simulink model "full_sim123deleteme"  (R2020b)
settings: Solver=ode1be  StartTime=0.0  StopTime=inf  RelTol=1e-3
InitFcn:
  | % Clear persistent variables in callback
  | clear all;
  | 
  | track = gen_track;
  | map = double(rgb2gray(imread('map.png')));%'iSpaceMapV2.0_50dpi.png')))*100/255;
  | 
  | % Load config data automatically
  | load("config.mat");
StartFcn:
  | % The event listener triggers when the signal updates, so we can just monitor one of the signals.
  | blk1 = 'full_sim/GUI_update';
  | 
  | event = 'PostOutputs';
  | listener = @updateApp;
  | 
  | % Create the listener
  | h1 = add_exec_event_listener(blk1, event, listener);
model workspace (MAT data in the model file):
  ResetMode = "Reset at each sample time"
  initX = -0.39
  initY = 0.33
  initYaw = 3.14159265359
libraries: simulink_extras x10, simulink x8, dspnetwork x6, pid_lib x2, sldrtlib x1
(part 1 of 2)
settings Model: Creator=Duncan  LastModifiedBy=dffleiss

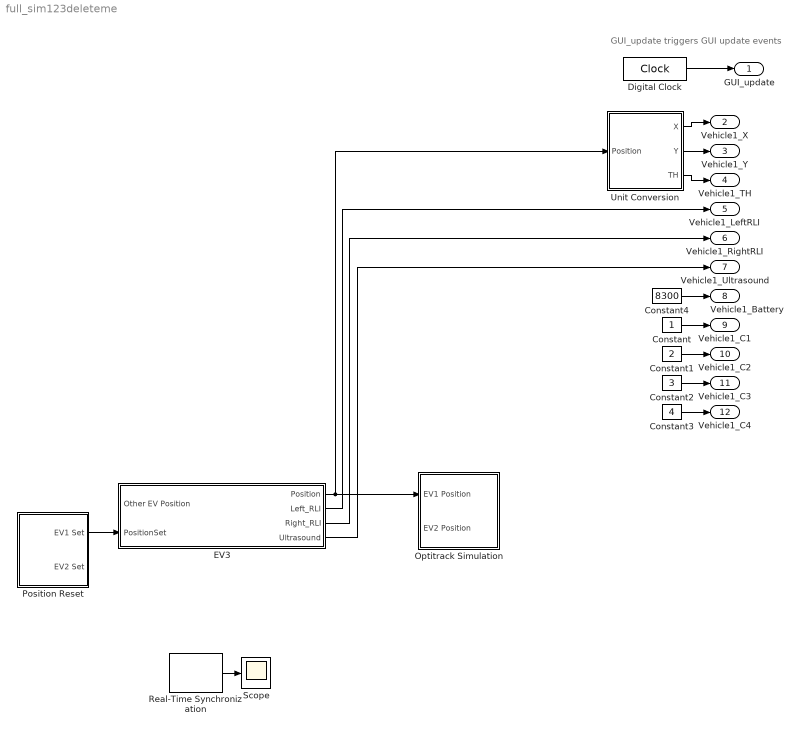
== system full_sim123deleteme ==
  note: GUI_update triggers GUI update events
  Constant : Constant
  Constant1 : Constant  Value=2
  Constant2 : Constant  Value=3
  Constant3 : Constant  Value=4
  Constant4 : Constant  Value=8300
  Digital Clock : DigitalClock  SampleTime=0.1
  EV3 : Subsystem
  Optitrack Simulation : Subsystem
  Position Reset : Subsystem
  Real-Time Synchronization : sldrtlib/Real-Time Synchronization  SampleTime=.01  MaxMissedTicks=inf  ShowMissedTicks=on  YieldWhenWaiting=off
  Scope : Scope
  Unit Conversion : Subsystem
  GUI_update : Outport
  Vehicle1_X : Outport  Port=2
  Vehicle1_Y : Outport  Port=3
  Vehicle1_TH : Outport  Port=4
  Vehicle1_LeftRLI : Outport  Port=5
  Vehicle1_RightRLI : Outport  Port=6
  Vehicle1_Ultrasound : Outport  Port=7
  Vehicle1_Battery : Outport  Port=8
  Vehicle1_C1 : Outport  Port=9
  Vehicle1_C2 : Outport  Port=10
  Vehicle1_C3 : Outport  Port=11
  Vehicle1_C4 : Outport  Port=12
  wires:
  Real-Time Synchronization/1 -> Scope/1
  Position Reset/1(EV1 Set) -> EV3/2(PositionSet)
  Constant2/1 -> Vehicle1_C3/1
  Constant4/1 -> Vehicle1_Battery/1
  Constant1/1 -> Vehicle1_C2/1
  EV3/2(Left_RLI) -> Vehicle1_LeftRLI/1
  Constant/1 -> Vehicle1_C1/1
  Constant3/1 -> Vehicle1_C4/1
  EV3/1(Position) -> Unit Conversion/1(Position), Optitrack Simulation/1(EV1 Position)
  Unit Conversion/2(Y) -> Vehicle1_Y/1
  Unit Conversion/3(TH) -> Vehicle1_TH/1
  Unit Conversion/1(X) -> Vehicle1_X/1
  Digital Clock/1 -> GUI_update/1
  EV3/3(Right_RLI) -> Vehicle1_RightRLI/1
  EV3/4(Ultrasound) -> Vehicle1_Ultrasound/1

== system full_sim123deleteme/EV3 ==
  Other EV Position : Inport
  PositionSet : Inport  Port=2
  Additive Noise : Subsystem
  Localization and UI Control : Subsystem
      settings: PortSchema="{\"entries\":[{\"content\":{\"sides\":[{\"content\":{\"connectorIds\":[\"Out1\",\"Out2\"]},\"type\":\"ConnectorPlacement.EquallySpacedRectSide\",\"uuid\":\"c41f9887-e70f-42cb-a70d-ce479c94e8e6\"},{\"content\":{\"connectorIds\":[\"In7\",\"In8\",\"In9\"],\"side\":\"RIGHT\"},\"type\":\"ConnectorPlacement.EquallySpacedRectSide\",\"uuid\":\"01fea69d-4e07-40c9-8b78-412f64609b36\"},{\"content\":{\"connectorIds\":[\"In1\",\"In2\",\"In3\",\"In4\",\"In5\",\"In6\"],\"side\":\"TOP\"},\"type\":\"ConnectorPlacement.EquallySpacedRectSide\",\"uuid\":\"d2fc7682-afac-46c9-9372-ea085883672c\"}]},\"type\":\"ConnectorPlacement.EquallySpacedConnector\",\"uuid\":\"f49fd9b7-3a1c-45a5-ac31-ef3904fd2313\"}],\"packageUris\":[\"http://schema.mathworks.com/mf0/Connector/19700101\"],\"version\":\"1.0\"}"
  Position Control : Subsystem
  Sensor Input Block : Subsystem
  Task Controls : Subsystem
      settings: PortSchema="{\"entries\":[{\"content\":{\"sides\":[{\"content\":{\"connectorIds\":[\"In1\",\"In2\",\"In3\",\"In4\",\"In5\"]},\"type\":\"ConnectorPlacement.EquallySpacedRectSide\",\"uuid\":\"3c64813c-625d-49d1-ae67-306451c3c1fa\"},{\"content\":{\"connectorIds\":[\"Out1\",\"Out2\",\"Out3\",\"Out4\"],\"side\":\"RIGHT\"},\"type\":\"ConnectorPlacement.EquallySpacedRectSide\",\"uuid\":\"91793cf5-b7a0-4d71-a2c0-83cdd43afca2\"},{\"content\":{\"connectorIds\":[],\"side\":\"TOP\"},\"type\":\"ConnectorPlacement.EquallySpacedRectSide\",\"uuid\":\"5300aefe-28d7-4142-9759-b53f625cf082\"},{\"content\":{\"connectorIds\":[\"Out5\",\"Out6\",\"Out7\",\"Out8\",\"Out9\",\"Out10\"],\"side\":\"BOTTOM\"},\"type\":\"ConnectorPlacement.EquallySpacedRectSide\",\"uuid\":\"7541b0a2-c079-4b1b-9276-8e4ee5949dfd\"},{\"content\":{\"connectorIds\":[],\"side\":\"HIDDEN\"},\"type\":\"ConnectorPlacement.EquallySpacedRectSide\",\"uuid\":\"d0ef4c96-52b1-4a81-ac1e-c57b650a37a1\"}]},\"type\":\"ConnectorPlacement.EquallySpacedConnector\",\"uuid\":\"d02aae7f-e4d5-4935-81ce-eef5c5855771\"}],\"packageUris\":[\"http://schema.mathworks.com/mf0/Connector/R2020b\"],\"version\":\"1.0\"}"
  Position : Outport
  Left_RLI : Outport  Port=2
  Right_RLI : Outport  Port=3
  Ultrasound : Outport  Port=4
  wires:
  Localization and UI Control/2(Left %) -> Task Controls/4(Left Motor %)
  Position Control/2(Gyro) -> Localization and UI Control/9(Gyro Rate (deg/s))
  Task Controls/2(Right Encoder) -> Localization and UI Control/8(Right Encoder (deg/sample))
  PositionSet/1 -> Position Control/1(Position Set)
  Other EV Position/1 -> Sensor Input Block/2(Other EV Position)
  Position Control/1(Position) -> Position/1, Sensor Input Block/1(Position)
  Localization and UI Control/1(Right %) -> Task Controls/5(Right Motor %)
  Task Controls/1(Left Encoder) -> Localization and UI Control/7(Left Encoder (deg/sample))
  Task Controls/4(Left ω) -> Position Control/3(Input1)
  Task Controls/3(Right ω) -> Position Control/2(Input)
  Task Controls/7(Speed) -> Localization and UI Control/3(LF Speed)
  Task Controls/6(Steering) -> Localization and UI Control/2(LF Steering)
  Task Controls/5(Platoon Speed) -> Localization and UI Control/1(Platoon Speed)
  Task Controls/10(Left RLI) -> Left_RLI/1, Localization and UI Control/6(Left RLI)
  Task Controls/9(Right RLI) -> Right_RLI/1, Localization and UI Control/5(Right RLI)
  Task Controls/8(Ultrasonic) -> Ultrasound/1, Localization and UI Control/4(Ultrasonic (cm))
  Sensor Input Block/1(Left RLI) -> Additive Noise/1(In1)
  Additive Noise/1(Out1) -> Task Controls/1(Left Input)
  Sensor Input Block/2(Right RLI) -> Additive Noise/2(In2)
  Sensor Input Block/3(Ultrasonic) -> Additive Noise/3(In3)
  Additive Noise/2(Out2) -> Task Controls/2(Right Input)
  Additive Noise/3(Out3) -> Task Controls/3(Distance Input)

== system full_sim123deleteme/Optitrack Simulation ==
  EV1 Position : Inport
  EV2 Position : Inport  Port=2
  MATLAB Function : MATLAB Function  TreatAsAtomicUnit=on
  UDP Send : dspnetwork/UDP Send  remoteURL='127.0.0.1'  remotePort=1511  localURL='0.0.0.0'  localPortSource=Automatically determine  localPort=-1  sendBufferSize=8192  sampletime=-1  blockPlatform=[]  separateLengthPort=0
  wires:
  EV1 Position/1 -> MATLAB Function/1(ev1pos)
  EV2 Position/1 -> MATLAB Function/2(ev2pos)
  MATLAB Function/1(packet) -> UDP Send/1

== system full_sim123deleteme/Position Reset ==
  AND : Logic  IconShape=distinctive  AllPortsSameDT=off  OutDataTypeStr=boolean
  AND1 : Logic  IconShape=distinctive  AllPortsSameDT=off  OutDataTypeStr=boolean
  Assignment : Assignment  DiagnosticForDimensions=Warning  IndexOptions=Index vector (dialog)  Indices=1  OutputSizes=1
  Assignment1 : Assignment  DiagnosticForDimensions=Warning  IndexOptions=Index vector (dialog)  Indices=1  OutputSizes=1
  Cast To Single : DataTypeConversion  OutDataTypeStr=single
  Cast To Single1 : DataTypeConversion  OutDataTypeStr=single
  Compare To Constant : simulink/Logic and Bit Operations/Compare To Constant  relop===  const=1  OutDataTypeStr=boolean
  Compare To Constant1 : simulink/Logic and Bit Operations/Compare To Constant  relop===  const=2  OutDataTypeStr=boolean
  Compare To Constant2 : simulink/Logic and Bit Operations/Compare To Constant  relop=>  const=0  OutDataTypeStr=boolean
  UDP Receive : dspnetwork/UDP Receive  localURL='0.0.0.0'  localPort=24999  remoteURL='0.0.0.0'  remotePort=-1  recvBufferSize=512  dims=4  signalDatatype=single  isComplex=off  isVarSize=off  showBlockingTime=off  blockingTime=0  sampletime=0.01  blockPlatform=[]
  ev : Selector  InputPortWidth=4  IndexOptions=Index vector (dialog)  Indices=[1]  OutputSizes=1
  EV1 Set : Outport
  EV2 Set : Outport  Port=2
  wires:
  Compare To Constant2/1 -> AND1/2, AND/2
  UDP Receive/2 -> Compare To Constant2/1
  ev/1 -> Compare To Constant1/1, Compare To Constant/1
  Assignment/1 -> EV1 Set/1
  Compare To Constant/1 -> AND1/1
  Assignment1/1 -> EV2 Set/1
  UDP Receive/1 -> Assignment/1, Assignment1/1, ev/1
  AND/1 -> Cast To Single1/1
  Compare To Constant1/1 -> AND/1
  Cast To Single/1 -> Assignment/2
  AND1/1 -> Cast To Single/1
  Cast To Single1/1 -> Assignment1/2

== system full_sim123deleteme/Unit Conversion ==
  Position : Inport
  Demux1 : Demux  Outputs=3
  Gain2 : Gain  Gain=1000
  Gain3 : Gain  Gain=1000
  MATLAB Function1 : MATLAB Function  TreatAsAtomicUnit=on
  Radians to Degrees1 : simulink_extras/Transformations/Radians to Degrees
  X : Outport
  Y : Outport  Port=2
  TH : Outport  Port=3
  wires:
  Radians to Degrees1/1 -> MATLAB Function1/1(u)
  Gain3/1 -> Y/1
  Demux1/3 -> Radians to Degrees1/1
  Demux1/2 -> Gain3/1
  Gain2/1 -> X/1
  MATLAB Function1/1(y) -> TH/1
  Demux1/1 -> Gain2/1
  Position/1 -> Demux1/1

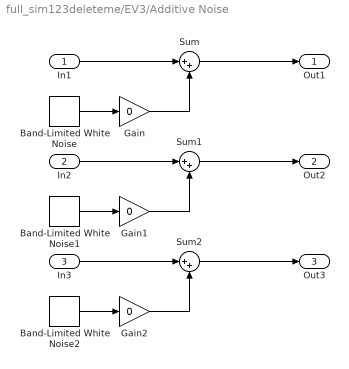
== system full_sim123deleteme/EV3/Additive Noise ==
  In1 : Inport
  In2 : Inport  Port=2
  In3 : Inport  Port=3
  Band-Limited White Noise : simulink/Sources/Band-Limited White Noise  Cov=[0.1]  Ts=0.1  seed=[23341]
  Band-Limited White Noise1 : simulink/Sources/Band-Limited White Noise  Cov=[0.1]  Ts=0.1  seed=[23341]
  Band-Limited White Noise2 : simulink/Sources/Band-Limited White Noise  Cov=[0.1]  Ts=0.1  seed=[23341]
  Gain : Gain  Gain=0
  Gain1 : Gain  Gain=0
  Gain2 : Gain  Gain=0
  Sum : Sum  Inputs=|++
  Sum1 : Sum  Inputs=|++
  Sum2 : Sum  Inputs=|++
  Out1 : Outport
  Out2 : Outport  Port=2
  Out3 : Outport  Port=3
  wires:
  In1/1 -> Sum/1
  Sum/1 -> Out1/1
  Band-Limited White Noise1/1 -> Gain1/1
  Sum1/1 -> Out2/1
  In2/1 -> Sum1/1
  Band-Limited White Noise2/1 -> Gain2/1
  Sum2/1 -> Out3/1
  In3/1 -> Sum2/1
  Band-Limited White Noise/1 -> Gain/1
  Gain/1 -> Sum/2
  Gain1/1 -> Sum1/2
  Gain2/1 -> Sum2/2

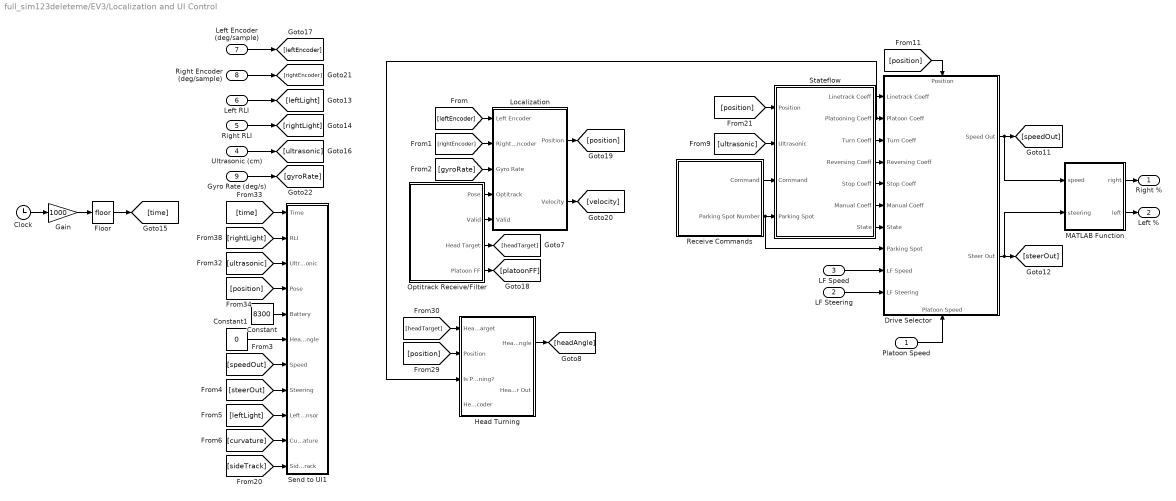
== system full_sim123deleteme/EV3/Localization and UI Control ==
  Platoon Speed : Inport
  LF Steering : Inport  Port=2
  LF Speed : Inport  Port=3
  Ultrasonic (cm) : Inport  Port=4
  Right RLI : Inport  Port=5
  Left RLI : Inport  Port=6
  Left Encoder (deg/sample) : Inport  Port=7
  Right Encoder (deg/sample) : Inport  Port=8
  Gyro Rate (deg/s) : Inport  Port=9
  Clock : Clock
  Constant : Constant  Value=8300
  Constant1 : Constant  Value=0
  Drive Selector : Subsystem
      settings: PortSchema="{\"entries\":[{\"content\":{\"sides\":[{\"content\":{\"connectorIds\":[\"In1\",\"In2\",\"In3\",\"In4\",\"In5\",\"In6\",\"In7\",\"In8\",\"In9\",\"In10\"]},\"type\":\"ConnectorPlacement.EquallySpacedRectSide\",\"uuid\":\"ae307232-287c-4602-bc59-e7aee20cf720\"},{\"content\":{\"connectorIds\":[\"Out1\",\"Out2\"],\"side\":\"RIGHT\"},\"type\":\"ConnectorPlacement.EquallySpacedRectSide\",\"uuid\":\"2cae2544-d808-4029-9530-a1f56251b9cd\"},{\"content\":{\"connectorIds\":[\"In11\"],\"side\":\"TOP\"},\"type\":\"ConnectorPlacement.EquallySpacedRectSide\",\"uuid\":\"bbc0be7b-0147-487e-824e-99eef1e06dcc\"},{\"content\":{\"connectorIds\":[\"In12\"],\"side\":\"BOTTOM\"},\"type\":\"ConnectorPlacement.EquallySpacedRectSide\",\"uuid\":\"b1fbed80-afe2-48db-af11-c85938407aae\"}]},\"type\":\"ConnectorPlacement.EquallySpacedConnector\",\"uuid\":\"38f7d747-6147-4f1b-8575-02c2e0fe0660\"}],\"packageUris\":[\"http://schema.mathworks.com/mf0/Connector/19700101\"],\"version\":\"1.0\"}"
  Floor : Rounding
  Gain : Gain  Gain=1000
  Head Turning : Subsystem
  Localization : Subsystem
  MATLAB Function : MATLAB Function  TreatAsAtomicUnit=on
  Optitrack Receive/Filter : Subsystem
  Receive Commands : Subsystem
  Send to UI1 : Subsystem
  Stateflow : Subsystem
  Right % : Outport
  Left % : Outport  Port=2
  wires:
  Constant/1 -> Send to UI1/5(Battery)
  [position] -> Head Turning/2(Position)
  Left RLI/1 -> [leftLight]
  Localization/2(Velocity) -> [velocity]
  Stateflow/6(Manual Coeff) -> Drive Selector/6(Manual Coeff)
  [leftEncoder] -> Localization/1(Left Encoder)
  MATLAB Function/1(right) -> Right %/1
  Head Turning/1(Head Angle) -> [headAngle]
  Optitrack Receive/Filter/4(Platoon FF) -> [platoonFF]
  [gyroRate] -> Localization/3(Gyro Rate)
  Floor/1 -> [time]
  Drive Selector/2(Steer Out) -> [steerOut], MATLAB Function/2(steering)
  Optitrack Receive/Filter/2(Valid) -> Localization/5(Valid)
  Clock/1 -> Gain/1
  Right Encoder (deg/sample)/1 -> [rightEncoder]
  Optitrack Receive/Filter/3(Head Target) -> [headTarget]
  Left Encoder (deg/sample)/1 -> [leftEncoder]
  Gain/1 -> Floor/1
  Receive Commands/1(Command) -> Stateflow/3(Command)
  [ultrasonic] -> Send to UI1/3(Ultrasonic)
  [curvature] -> Send to UI1/10(Curvature)
  Stateflow/4(Reversing Coeff) -> Drive Selector/4(Reversing Coeff)
  Gyro Rate (deg/s)/1 -> [gyroRate]
  [leftLight] -> Send to UI1/9(Left Sensor)
  [sideTrack] -> Send to UI1/11(Side Track)
  Drive Selector/1(Speed Out) -> [speedOut], MATLAB Function/1(speed)
  Right RLI/1 -> [rightLight]
  Ultrasonic (cm)/1 -> [ultrasonic]
  MATLAB Function/2(left) -> Left %/1
  [speedOut] -> Send to UI1/7(Speed)
  [steerOut] -> Send to UI1/8(Steering)
  Stateflow/7(State) -> Drive Selector/7(State)
  Stateflow/5(Stop Coeff) -> Drive Selector/5(Stop Coeff)
  Localization/1(Position) -> [position]
  Optitrack Receive/Filter/1(Pose) -> Localization/4(Optitrack)
  [position] -> Send to UI1/4(Pose)
  Stateflow/3(Turn Coeff) -> Drive Selector/3(Turn Coeff)
  [rightLight] -> Send to UI1/2(RLI)
  Stateflow/2(Platooning Coeff) -> Head Turning/3(Is Platooning?), Drive Selector/2(Platoon Coeff)
  [ultrasonic] -> Stateflow/2(Ultrasonic)
  [headTarget] -> Head Turning/1(Head Target)
  [position] -> Stateflow/1(Position)
  Stateflow/1(Linetrack Coeff) -> Drive Selector/1(Linetrack Coeff)
  Receive Commands/2(Parking Spot Number) -> Drive Selector/8(Parking Spot), Stateflow/4(Parking Spot)
  [position] -> Drive Selector/11(Position)
  [rightEncoder] -> Localization/2(Right Encoder)
  [time] -> Send to UI1/1(Time)
  Constant1/1 -> Send to UI1/6(Head Angle)
  LF Speed/1 -> Drive Selector/9(LF Speed)
  LF Steering/1 -> Drive Selector/10(LF Steering)
  Platoon Speed/1 -> Drive Selector/12(Platoon Speed)

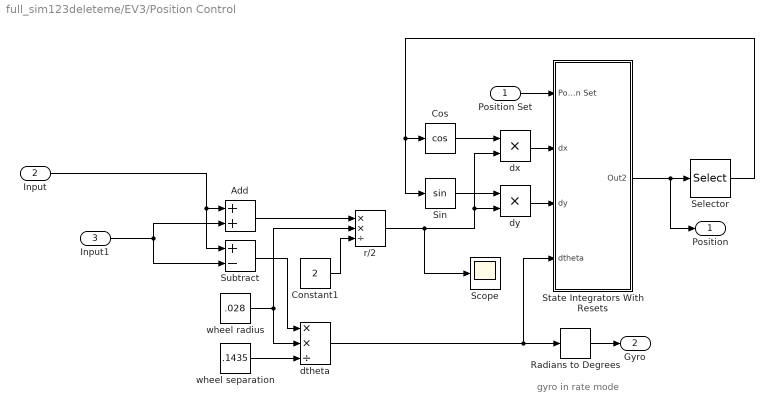
== system full_sim123deleteme/EV3/Position Control ==
  note: gyro in rate mode
  Position Set : Inport
  Input : Inport  Port=2
  Input1 : Inport  Port=3
  Add : Sum
  Constant1 : Constant  Value=2
  Cos : Trigonometry  Operator=cos
  Radians to Degrees : simulink_extras/Transformations/Radians to Degrees
  Scope : Scope
  Selector : Selector  InputPortWidth=3  IndexOptions=Index vector (dialog)  Indices=3  OutputSizes=1
  Sin : Trigonometry
  State Integrators With Resets : Subsystem
  Subtract : Sum  Inputs=+-
  dtheta : Product  Inputs=**/
  dx : Product  Inputs=**
  dy : Product  Inputs=**
  r/2 : Product  Inputs=**/
  wheel radius : Constant  Value=.028
  wheel separation : Constant  Value=.1435
  Position : Outport
  Gyro : Outport  Port=2
  wires:
  Position Set/1 -> State Integrators With Resets/1(Position Set)
  Input/1 -> Add/1, Subtract/1
  State Integrators With Resets/1(Out2) -> Selector/1, Position/1
  dtheta/1 -> State Integrators With Resets/4(dtheta), Radians to Degrees/1
  Input1/1 -> Add/2, Subtract/2
  Cos/1 -> dx/1
  dy/1 -> State Integrators With Resets/3(dy)
  dx/1 -> State Integrators With Resets/2(dx)
  r/2/1 -> Scope/1, dx/2, dy/2
  wheel separation/1 -> dtheta/3
  Selector/1 -> Cos/1, Sin/1
  wheel radius/1 -> r/2/2, dtheta/2
  Subtract/1 -> dtheta/1
  Sin/1 -> dy/1
  Add/1 -> r/2/1
  Radians to Degrees/1 -> Gyro/1
  Constant1/1 -> r/2/3

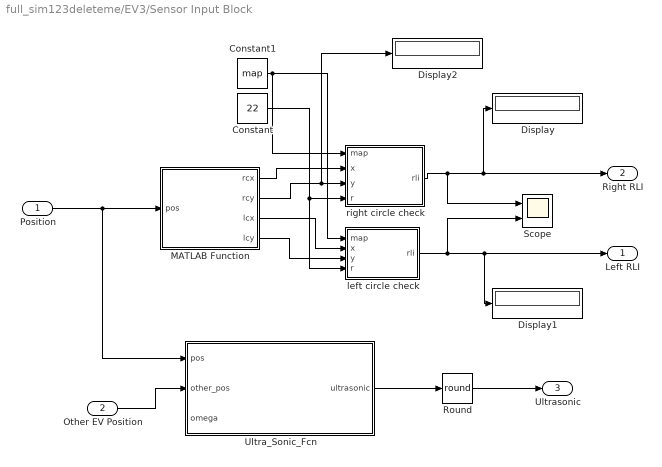
== system full_sim123deleteme/EV3/Sensor Input Block ==
  Position : Inport
  Other EV Position : Inport  Port=2
  Constant : Constant  Value=22
  Constant1 : Constant  Value=map
  Display : Display
  Display1 : Display
  Display2 : Display
  MATLAB Function : MATLAB Function  TreatAsAtomicUnit=on
  Round : Rounding  Operator=round
  Scope : Scope  NumInputPorts=2
  Ultra_Sonic_Fcn : MATLAB Function  TreatAsAtomicUnit=on
  left circle check : MATLAB Function  TreatAsAtomicUnit=on
  right circle check : MATLAB Function  TreatAsAtomicUnit=on
  Left RLI : Outport
  Right RLI : Outport  Port=2
  Ultrasonic : Outport  Port=3
  wires:
  Constant/1 -> right circle check/4(r), left circle check/4(r)
  MATLAB Function/4(lcy) -> left circle check/3(y)
  MATLAB Function/3(lcx) -> left circle check/2(x)
  Position/1 -> Ultra_Sonic_Fcn/1(pos), MATLAB Function/1(pos)
  Constant1/1 -> left circle check/1(map), right circle check/1(map)
  MATLAB Function/2(rcy) -> Display2/1, right circle check/3(y)
  MATLAB Function/1(rcx) -> right circle check/2(x)
  right circle check/1(rli) -> Display/1, Right RLI/1, Scope/1
  left circle check/1(rli) -> Display1/1, Left RLI/1, Scope/2
  Other EV Position/1 -> Ultra_Sonic_Fcn/2(other_pos)
  Round/1 -> Ultrasonic/1
  Ultra_Sonic_Fcn/1(ultrasonic) -> Round/1

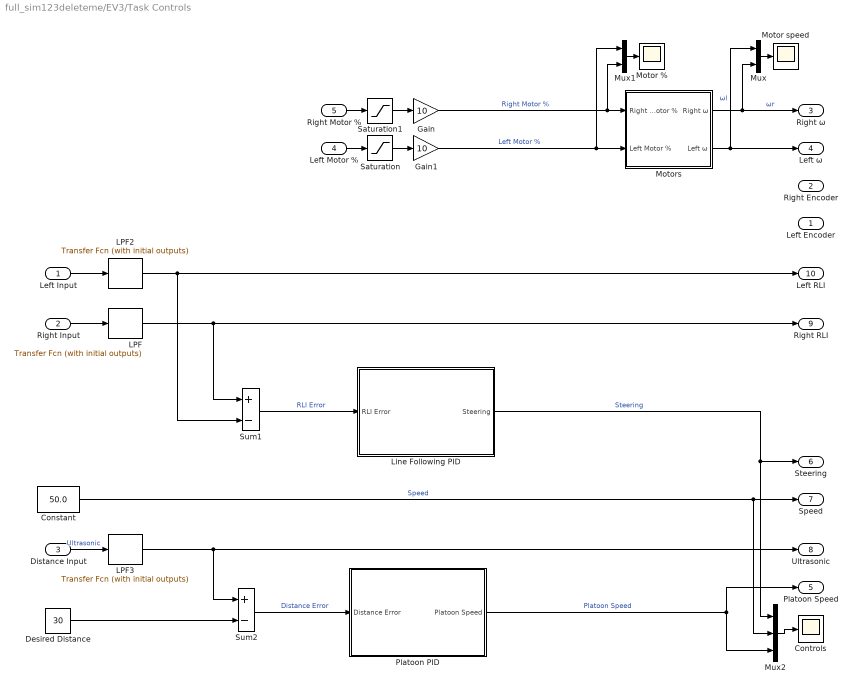
== system full_sim123deleteme/EV3/Task Controls ==
  Left Input : Inport
  Right Input : Inport  Port=2
  Distance Input : Inport  Port=3
  Left Motor % : Inport  Port=4
  Right Motor % : Inport  Port=5
  Constant : Constant  Value=50.0
  Controls : Scope
  Desired Distance : Constant  Value=30
  Gain : Gain  Gain=10
  Gain1 : Gain  Gain=10
  LPF : simulink_extras/Additional Linear/Transfer Fcn (with initial outputs)  N=[1]  D="[0.02  1]"  Y0=0  U0=0
  LPF2 : simulink_extras/Additional Linear/Transfer Fcn (with initial outputs)  N=[1]  D="[0.02  1]"  Y0=0  U0=0
  LPF3 : simulink_extras/Additional Linear/Transfer Fcn (with initial outputs)  N=[1]  D="[0.02  1]"  Y0=0  U0=0
  Line Following PID : Subsystem
  Motor % : Scope
  Motor speed : Scope
  Motors : Subsystem
  Mux : Mux  Inputs=2
  Mux1 : Mux  Inputs=2
  Mux2 : Mux  Inputs=3
  Platoon PID : Subsystem
  Saturation : Saturate  UpperLimit=100  LowerLimit=-100
  Saturation1 : Saturate  UpperLimit=100  LowerLimit=-100
  Sum1 : Sum  Inputs=+-
  Sum2 : Sum  Inputs=+-
  Left Encoder : Outport
  Right Encoder : Outport  Port=2
  Right ω : Outport  Port=3
  Left ω : Outport  Port=4
  Platoon Speed : Outport  Port=5
  Steering : Outport  Port=6
  Speed : Outport  Port=7
  Ultrasonic : Outport  Port=8
  Right RLI : Outport  Port=9
  Left RLI : Outport  Port=10
  wires:
  LPF2/1 -> Sum1/2, Left RLI/1
  Motors/1(Right ω) -> Mux/2, Right ω/1  "ωr"
  Motors/2(Left ω) -> Mux/1, Left ω/1  "ωl"
  Mux/1 -> Motor speed/1
  Mux1/1 -> Motor %/1
  Gain/1 -> Mux1/2, Motors/1(Right Motor %)  "Right Motor %"
  Gain1/1 -> Mux1/1, Motors/2(Left Motor %)  "Left Motor %"
  Constant/1 -> Mux2/2, Speed/1  "Speed"
  Left Motor %/1 -> Saturation/1
  Right Motor %/1 -> Saturation1/1
  Mux2/1 -> Controls/1
  Right Input/1 -> LPF/1
  LPF/1 -> Sum1/1, Right RLI/1
  Left Input/1 -> LPF2/1
  Saturation/1 -> Gain1/1
  Saturation1/1 -> Gain/1
  Distance Input/1 -> LPF3/1  "Ultrasonic"
  Desired Distance/1 -> Sum2/2
  LPF3/1 -> Sum2/1, Ultrasonic/1
  Platoon PID/1(Platoon Speed) -> Mux2/3, Platoon Speed/1  "Platoon Speed"
  Sum2/1 -> Platoon PID/1(Distance Error)  "Distance Error"
  Line Following PID/1(Steering) -> Mux2/1, Steering/1  "Steering"
  Sum1/1 -> Line Following PID/1(RLI Error)  "RLI Error"

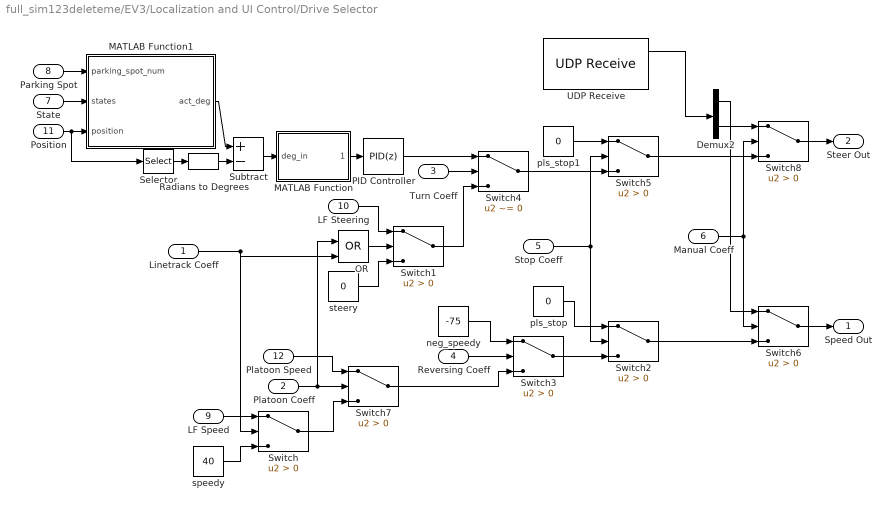
== system full_sim123deleteme/EV3/Localization and UI Control/Drive Selector ==
  Linetrack Coeff : Inport
  Platoon Coeff : Inport  Port=2
  Turn Coeff : Inport  Port=3
  Reversing Coeff : Inport  Port=4
  Stop Coeff : Inport  Port=5
  Manual Coeff : Inport  Port=6
  State : Inport  Port=7
  Parking Spot : Inport  Port=8
  LF Speed : Inport  Port=9
  LF Steering : Inport  Port=10
  Position : Inport  Port=11
  Platoon Speed : Inport  Port=12
  Demux2 : Demux  Outputs=2
  MATLAB Function : MATLAB Function  TreatAsAtomicUnit=on
  MATLAB Function1 : MATLAB Function  TreatAsAtomicUnit=on
  OR : Logic  Operator=OR  IconShape=distinctive  AllPortsSameDT=off  OutDataTypeStr=boolean
  PID Controller : pid_lib/PID Controller  Controller=PID  Form=Parallel  TimeDomain=Discrete-time  UseExternalTs=off  SampleTime=-1  IntegratorMethod=Forward Euler  FilterMethod=Forward Euler  ControllerParametersSource=internal  P=1  I=0  D=0  UseFilter=off  N=100  TunerSelectOption=Transfer Function Based (PID Tuner App)  InitialConditionSource=internal  InitialConditionForIntegrator=0  InitialConditionForFilter=0  DifferentiatorICPrevScaledInput=0  ExternalReset=none  TrackingMode=off  Kt=1  LimitOutput=off  SatLimitsSource=internal  UpperSaturationLimit=inf  LowerSaturationLimit=-inf  LinearizeAsGain=on  AntiWindupMode=none  Kb=1  POutMin=[]  POutMax=[]  IOutMin=[]  IOutMax=[]  DOutMin=[]  DOutMax=[]  NOutMin=[]  NOutMax=[]  SumOutMin=[]  SumOutMax=[]  SaturationOutMin=[]  SaturationOutMax=[]  PParamMin=[]  PParamMax=[]  IParamMin=[]  IParamMax=[]  DParamMin=[]  DParamMax=[]  NParamMin=[]  NParamMax=[]  KbParamMin=[]  KbParamMax=[]  KtParamMin=[]  KtParamMax=[]  KbOutMin=[]  KbOutMax=[]  KtOutMin=[]  KtOutMax=[]  IntegratorOutMin=[]  IntegratorOutMax=[]  FilterOutMin=[]  FilterOutMax=[]  SumI1OutMin=[]  SumI1OutMax=[]  SumI2OutMin=[]  SumI2OutMax=[]  SumI3OutMin=[]  SumI3OutMax=[]  SumI4OutMin=[]  SumI4OutMax=[]  SumDOutMin=[]  SumDOutMax=[]  DifferentiatorOutMin=[]  DifferentiatorOutMax=[]  FilterDiffOutCoefMin=[]  FilterDiffOutCoefMax=[]  ReciprocalOutMin=[]  ReciprocalOutMax=[]  SumDenOutMin=[]  SumDenOutMax=[]  SumNumOutMin=[]  SumNumOutMax=[]  DivideOutMin=[]  DivideOutMax=[]  UdiffTsProdOutMin=[]  UdiffTsProdOutMax=[]  NTsProdOutMin=[]  NTsProdOutMax=[]  UintegralTsProdOutMin=[]  UintegralTsProdOutMax=[]  UngainTsProdOutMin=[]  UngainTsProdOutMax=[]  IntegratorContinuousStateAttributes=''  IntegratorStateMustResolveToSignalObject=off  IntegratorRTWStateStorageClass=Auto  FilterContinuousStateAttributes=''  FilterStateMustResolveToSignalObject=off  FilterRTWStateStorageClass=Auto  ParallelPVariant=InternalParameters  IdealPVariant=Disabled  IVariant=InternalParameters  DVariant=InternalParameters  IntegratorVariant=Discrete  SatVariant=Disabled  AWVariant=Passthrough  PCopyVariant=Disabled  TRVariant=Disabled  FdbkBlocksVariant=Forward  IdealPFdbkVariant=Disabled  SatFdbkVariant=Disabled  DerivativeFilterVariant=Differentiator  NVariant=Passthrough  NCopyVariant=Disabled_SignalSpec  FilterICVariant=InternalICsDifferentiator  IntegratorICVariant=InternalICs  ExternalResetVariant=Disabled  TRSumVariant=Passthrough  SumFdbkVariant=Disabled  SumVariant=Sum_PID  TsampFilterVariant=InternalTs  TsampNgainVariant=Passthrough  TsampIntegralVariant=Passthrough  ExternalSaturationOutDataTypeStr=Inherit: Same as second input
  Radians to Degrees : simulink_extras/Transformations/Radians to Degrees
  Selector : Selector  InputPortWidth=3  IndexOptions=Index vector (dialog)  Indices=[3]  OutputSizes=1
  Subtract : Sum  Inputs=+-
  Switch{,1..3,5..8} (8 alike) : Switch  Criteria=u2 > Threshold
  Switch4 : Switch  Criteria=u2 ~= 0
  UDP Receive : dspnetwork/UDP Receive  localURL='0.0.0.0'  localPort=joystickRXPort  remoteURL='0.0.0.0'  remotePort=-1  recvBufferSize=384  dims=2  signalDatatype=single  isComplex=off  isVarSize=off  showBlockingTime=off  blockingTime=0  sampletime=0.01  blockPlatform=[]
  neg_speedy : Constant  Value=-75
  pls_stop : Constant  Value=0
  pls_stop1 : Constant  Value=0
  speedy : Constant  Value=40
  steery : Constant  Value=0
  Speed Out : Outport
  Steer Out : Outport  Port=2
  wires:
  Demux2/1 -> Switch6/1
  Demux2/2 -> Switch8/1
  Switch6/1 -> Speed Out/1
  Switch8/1 -> Steer Out/1
  Manual Coeff/1 -> Switch6/2, Switch8/2
  Switch2/1 -> Switch6/3
  Switch5/1 -> Switch8/3
  UDP Receive/1 -> Demux2/1
  LF Speed/1 -> Switch/1
  LF Steering/1 -> Switch1/1
  steery/1 -> Switch1/3
  speedy/1 -> Switch/3
  Switch1/1 -> Switch4/3
  Switch3/1 -> Switch2/3
  Stop Coeff/1 -> Switch2/2, Switch5/2
  pls_stop/1 -> Switch2/1
  Turn Coeff/1 -> Switch4/2
  PID Controller/1 -> Switch4/1
  Subtract/1 -> MATLAB Function/1(deg_in)
  MATLAB Function/1(deg_out) -> PID Controller/1
  Radians to Degrees/1 -> Subtract/2
  Parking Spot/1 -> MATLAB Function1/1(parking_spot_num)
  Reversing Coeff/1 -> Switch3/2
  State/1 -> MATLAB Function1/2(states)
  Position/1 -> Selector/1, MATLAB Function1/3(position)
  Switch4/1 -> Switch5/3
  neg_speedy/1 -> Switch3/1
  MATLAB Function1/1(act_deg) -> Subtract/1
  OR/1 -> Switch1/2
  Platoon Coeff/1 -> OR/1, Switch7/2
  Linetrack Coeff/1 -> Switch/2, OR/2
  Switch7/1 -> Switch3/3
  Switch/1 -> Switch7/3
  Selector/1 -> Radians to Degrees/1
  pls_stop1/1 -> Switch5/1
  Platoon Speed/1 -> Switch7/1

== system full_sim123deleteme/EV3/Localization and UI Control/Head Turning ==
  Head Target : Inport
  Position : Inport  Port=2
  Is Platooning? : Inport  Port=3
  Head Encoder : Inport  Port=4
  Discrete PID Controller : pid_lib/PID Controller  Controller=PID  Form=Parallel  TimeDomain=Discrete-time  UseExternalTs=off  SampleTime=-1  IntegratorMethod=Forward Euler  FilterMethod=Forward Euler  ControllerParametersSource=internal  P=1  I=1  D=0  UseFilter=off  N=100  TunerSelectOption=Transfer Function Based (PID Tuner App)  InitialConditionSource=internal  InitialConditionForIntegrator=0  InitialConditionForFilter=0  DifferentiatorICPrevScaledInput=0  ExternalReset=none  TrackingMode=off  Kt=1  LimitOutput=off  SatLimitsSource=internal  UpperSaturationLimit=inf  LowerSaturationLimit=-inf  LinearizeAsGain=off  AntiWindupMode=none  Kb=1  POutMin=[]  POutMax=[]  IOutMin=[]  IOutMax=[]  DOutMin=[]  DOutMax=[]  NOutMin=[]  NOutMax=[]  SumOutMin=[]  SumOutMax=[]  SaturationOutMin=[]  SaturationOutMax=[]  PParamMin=[]  PParamMax=[]  IParamMin=[]  IParamMax=[]  DParamMin=[]  DParamMax=[]  NParamMin=[]  NParamMax=[]  KbParamMin=[]  KbParamMax=[]  KtParamMin=[]  KtParamMax=[]  KbOutMin=[]  KbOutMax=[]  KtOutMin=[]  KtOutMax=[]  IntegratorOutMin=[]  IntegratorOutMax=[]  FilterOutMin=[]  FilterOutMax=[]  SumI1OutMin=[]  SumI1OutMax=[]  SumI2OutMin=[]  SumI2OutMax=[]  SumI3OutMin=[]  SumI3OutMax=[]  SumI4OutMin=[]  SumI4OutMax=[]  SumDOutMin=[]  SumDOutMax=[]  DifferentiatorOutMin=[]  DifferentiatorOutMax=[]  FilterDiffOutCoefMin=[]  FilterDiffOutCoefMax=[]  ReciprocalOutMin=[]  ReciprocalOutMax=[]  SumDenOutMin=[]  SumDenOutMax=[]  SumNumOutMin=[]  SumNumOutMax=[]  DivideOutMin=[]  DivideOutMax=[]  UdiffTsProdOutMin=[]  UdiffTsProdOutMax=[]  NTsProdOutMin=[]  NTsProdOutMax=[]  UintegralTsProdOutMin=[]  UintegralTsProdOutMax=[]  UngainTsProdOutMin=[]  UngainTsProdOutMax=[]  IntegratorContinuousStateAttributes=''  IntegratorStateMustResolveToSignalObject=off  IntegratorRTWStateStorageClass=Auto  FilterContinuousStateAttributes=''  FilterStateMustResolveToSignalObject=off  FilterRTWStateStorageClass=Auto  ParallelPVariant=InternalParameters  IdealPVariant=Disabled  IVariant=InternalParameters  DVariant=InternalParameters  IntegratorVariant=Discrete  SatVariant=Disabled  AWVariant=Passthrough  PCopyVariant=Disabled  TRVariant=Disabled  FdbkBlocksVariant=Forward  IdealPFdbkVariant=Disabled  SatFdbkVariant=Disabled  DerivativeFilterVariant=Differentiator  NVariant=Passthrough  NCopyVariant=Disabled_SignalSpec  FilterICVariant=InternalICsDifferentiator  IntegratorICVariant=InternalICs  ExternalResetVariant=Disabled  TRSumVariant=Passthrough  SumFdbkVariant=Disabled  SumVariant=Sum_PID  TsampFilterVariant=InternalTs  TsampNgainVariant=Passthrough  TsampIntegralVariant=Passthrough  ExternalSaturationOutDataTypeStr=Inherit: Same as second input
  MATLAB Function : MATLAB Function  TreatAsAtomicUnit=on
  Sum5 : Sum  Inputs=+|-
  Switch : Switch  Criteria=u2 > Threshold
  Zero1 : Constant  Value=0  OutDataTypeStr=Inherit: Inherit via back propagation
  Head Angle : Outport
  Head Motor Out : Outport  Port=2
  wires:
  Head Encoder/1 -> Sum5/2
  Position/1 -> MATLAB Function/2(position)
  Sum5/1 -> Discrete PID Controller/1
  Zero1/1 -> Switch/3
  Switch/1 -> Head Angle/1, Sum5/1
  Discrete PID Controller/1 -> Head Motor Out/1
  Head Target/1 -> MATLAB Function/1(headTarget)
  MATLAB Function/1(angle) -> Switch/1
  Is Platooning?/1 -> Switch/2

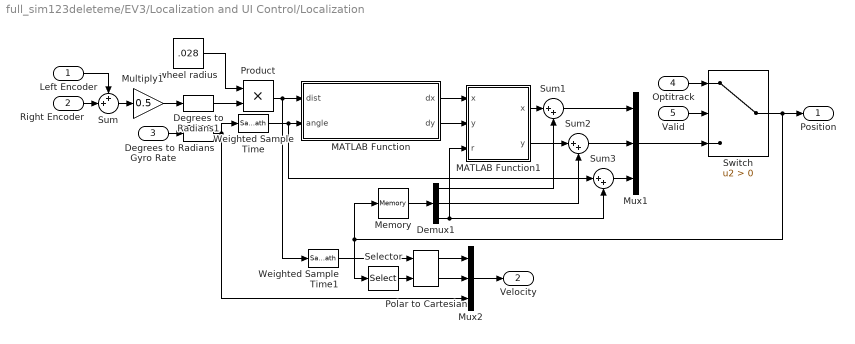
== system full_sim123deleteme/EV3/Localization and UI Control/Localization ==
  Left Encoder : Inport
  Right Encoder : Inport  Port=2
  Gyro Rate : Inport  Port=3
  Optitrack : Inport  Port=4
  Valid : Inport  Port=5
  Degrees to Radians : simulink_extras/Transformations/Degrees to Radians
  Degrees to Radians1 : simulink_extras/Transformations/Degrees to Radians
  Demux1 : Demux  Outputs=3
  MATLAB Function : MATLAB Function  TreatAsAtomicUnit=on
  MATLAB Function1 : MATLAB Function  TreatAsAtomicUnit=on
  Memory : Memory
  Multiply1 : Gain  Gain=0.5
  Mux1 : Mux  Inputs=3
  Mux2 : Mux  Inputs=3
  Polar to Cartesian : simulink_extras/Transformations/Polar to Cartesian
      settings: SourceProductBaseCode=SL
  Product : Product
  Selector : Selector  InputPortWidth=3  IndexOptions=Index vector (dialog)  Indices=[3]  OutputSizes=1
  Sum : Sum  Inputs=++|
  Sum1 : Sum  Inputs=|++
  Sum2 : Sum  Inputs=|++
  Sum3 : Sum  Inputs=|++
  Switch : Switch  Criteria=u2 > Threshold
  Weighted Sample Time : SampleTimeMath  TsampMathOp=*
  Weighted Sample Time1 : SampleTimeMath  TsampMathOp=/
  wheel radius : Constant  Value=.028
  Position : Outport
  Velocity : Outport  Port=2
  wires:
  Sum/1 -> Multiply1/1
  MATLAB Function/1(dx) -> MATLAB Function1/1("x ")
  MATLAB Function/2(dy) -> MATLAB Function1/2("y ")
  Memory/1 -> Demux1/1
  Demux1/3 -> MATLAB Function1/3(r), Sum3/2
  MATLAB Function1/1(x) -> Sum1/1
  MATLAB Function1/2(y) -> Sum2/1
  Demux1/1 -> Sum1/2
  Demux1/2 -> Sum2/2
  Sum1/1 -> Mux1/1
  Sum2/1 -> Mux1/2
  Sum3/1 -> Mux1/3
  Left Encoder/1 -> Sum/1
  Right Encoder/1 -> Sum/2
  Gyro Rate/1 -> Degrees to Radians/1
  Degrees to Radians/1 -> Mux2/3, Weighted Sample Time/1
  Weighted Sample Time/1 -> Sum3/1, MATLAB Function/2(angle)
  Mux1/1 -> Switch/3
  Valid/1 -> Switch/2
  Optitrack/1 -> Switch/1
  Switch/1 -> Position/1, Memory/1, Selector/1
  Selector/1 -> Polar to Cartesian/2
  Polar to Cartesian/1 -> Mux2/1
  Polar to Cartesian/2 -> Mux2/2
  Mux2/1 -> Velocity/1
  Weighted Sample Time1/1 -> Polar to Cartesian/1
  Multiply1/1 -> Degrees to Radians1/1
  Product/1 -> Weighted Sample Time1/1, MATLAB Function/1(dist)
  Degrees to Radians1/1 -> Product/2
  wheel radius/1 -> Product/1

== system full_sim123deleteme/EV3/Localization and UI Control/Optitrack Receive//Filter ==
  MATLAB Function : MATLAB Function  TreatAsAtomicUnit=on
  Memory : Memory
  Memory1 : Memory
  Scope : Scope
  Selector : Selector  InputPortWidth=6  IndexOptions=Index vector (dialog)  Indices=[1:3]  OutputSizes=1
  Selector1 : Selector  InputPortWidth=6  IndexOptions=Index vector (dialog)  Indices=[4:6]  OutputSizes=1
  Selector2 : Selector  InputPortWidth=3  IndexOptions=Index vector (dialog)  Indices=[1:2]  OutputSizes=1
  Selector3 : Selector  InputPortWidth=3  IndexOptions=Index vector (dialog)  Indices=[3]  OutputSizes=1
  Switch : Switch  Criteria=u2 > Threshold
  UDP Receive : dspnetwork/UDP Receive  localURL='0.0.0.0'  localPort=dataRXPort  remoteURL='0.0.0.0'  remotePort=-1  recvBufferSize=384  dims=6  signalDatatype=single  isComplex=off  isVarSize=off  showBlockingTime=off  blockingTime=0  sampletime=0.01  blockPlatform=[]
  Pose : Outport
  Valid : Outport  Port=2
  Head Target : Outport  Port=3
  Platoon FF : Outport  Port=4
  wires:
  MATLAB Function/1(valid) -> Valid/1
  MATLAB Function/2(arr) -> Memory1/1
  Memory1/1 -> MATLAB Function/3("arr ")
  Selector/1 -> Pose/1, MATLAB Function/1(data)
  Memory/1 -> Switch/3
  Switch/1 -> Selector2/1, Selector3/1, Memory/1
  Selector1/1 -> Switch/1
  UDP Receive/1 -> Selector/1, Selector1/1
  Selector2/1 -> Head Target/1
  Selector3/1 -> Platoon FF/1
  UDP Receive/2 -> Scope/1, Switch/2, MATLAB Function/2(new)

== system full_sim123deleteme/EV3/Localization and UI Control/Receive Commands ==
  Delay : Delay  DelayLength=1  InitialCondition=0
  Delay1 : Delay  DelayLength=1  InitialCondition=0
  Demux : Demux  Outputs=2
  Switch : Switch  Threshold=1
  Switch1 : Switch  Threshold=2
  UDP Receive : dspnetwork/UDP Receive  localURL='0.0.0.0'  localPort=cmdPort  remoteURL='0.0.0.0'  remotePort=-1  recvBufferSize=384  dims=2  signalDatatype=uint8  isComplex=off  isVarSize=off  showBlockingTime=off  blockingTime=0  sampletime=0.01  blockPlatform=[]
  Command : Outport
  Parking Spot Number : Outport  Port=2
  wires:
  UDP Receive/2 -> Switch/2, Switch1/2
  UDP Receive/1 -> Demux/1
  Demux/1 -> Switch/1
  Switch/1 -> Command/1, Delay/1
  Delay/1 -> Switch/3
  Switch1/1 -> Parking Spot Number/1, Delay1/1
  Delay1/1 -> Switch1/3
  Demux/2 -> Switch1/1

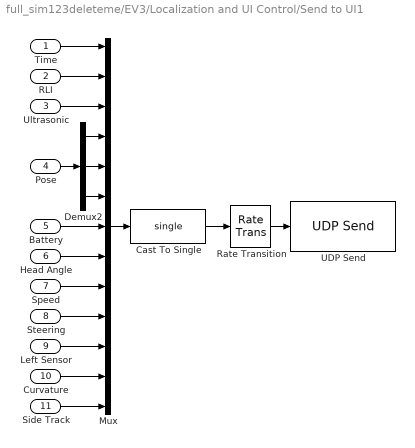
== system full_sim123deleteme/EV3/Localization and UI Control/Send to UI1 ==
  Time : Inport
  RLI : Inport  Port=2
  Ultrasonic : Inport  Port=3
  Pose : Inport  Port=4
  Battery : Inport  Port=5
  Head Angle : Inport  Port=6
  Speed : Inport  Port=7
  Steering : Inport  Port=8
  Left Sensor : Inport  Port=9
  Curvature : Inport  Port=10
  Side Track : Inport  Port=11
  Cast To Single : DataTypeConversion  OutDataTypeStr=single
  Demux2 : Demux  Outputs=3
  Mux : Mux  Inputs=13
  Rate Transition : RateTransition  OutPortSampleTime=.04
  UDP Send : dspnetwork/UDP Send  remoteURL='127.0.0.1'  remotePort=dataTXPort  localURL='0.0.0.0'  localPortSource=Automatically determine  localPort=-1  sendBufferSize=8192  sampletime=-1  blockPlatform=[]  separateLengthPort=0
  wires:
  Rate Transition/1 -> UDP Send/1
  Demux2/1 -> Mux/4
  Ultrasonic/1 -> Mux/3
  Pose/1 -> Demux2/1
  Battery/1 -> Mux/7
  Mux/1 -> Cast To Single/1
  Demux2/2 -> Mux/5
  Demux2/3 -> Mux/6
  RLI/1 -> Mux/2
  Cast To Single/1 -> Rate Transition/1
  Time/1 -> Mux/1
  Speed/1 -> Mux/9
  Head Angle/1 -> Mux/8
  Steering/1 -> Mux/10
  Left Sensor/1 -> Mux/11
  Curvature/1 -> Mux/12
  Side Track/1 -> Mux/13

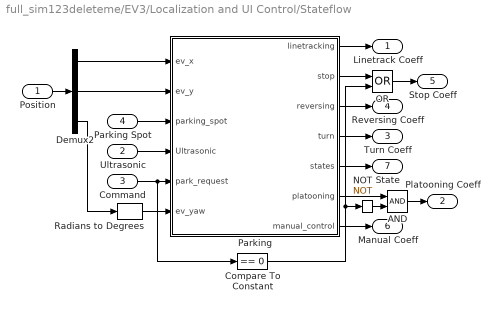
== system full_sim123deleteme/EV3/Localization and UI Control/Stateflow ==
  Position : Inport
  Ultrasonic : Inport  Port=2
  Command : Inport  Port=3
  Parking Spot : Inport  Port=4
  AND : Logic  IconShape=distinctive  AllPortsSameDT=off  OutDataTypeStr=boolean
  Compare To Constant : simulink/Logic and Bit Operations/Compare To Constant  relop===  const=0  OutDataTypeStr=boolean
  Demux2 : Demux  Outputs=3
  NOT : Logic  Operator=NOT  IconShape=distinctive  AllPortsSameDT=off  OutDataTypeStr=boolean
  OR : Logic  Operator=OR  IconShape=distinctive  AllPortsSameDT=off  OutDataTypeStr=boolean
  Parking : Stateflow chart  TreatAsAtomicUnit=on
  Radians to Degrees : simulink_extras/Transformations/Radians to Degrees
  Linetrack Coeff : Outport
  Platooning Coeff : Outport  Port=2
  Turn Coeff : Outport  Port=3
  Reversing Coeff : Outport  Port=4
  Stop Coeff : Outport  Port=5
  Manual Coeff : Outport  Port=6
  State : Outport  Port=7
  wires:
  NOT/1 -> AND/2
  AND/1 -> Platooning Coeff/1
  Parking/6(platooning) -> AND/1
  Compare To Constant/1 -> OR/2, NOT/1
  Parking/2(stop) -> OR/1
  OR/1 -> Stop Coeff/1
  Parking/7(manual_control) -> Manual Coeff/1
  Demux2/3 -> Radians to Degrees/1
  Ultrasonic/1 -> Parking/4(Ultrasonic)
  Parking/1(linetracking) -> Linetrack Coeff/1
  Demux2/2 -> Parking/2(ev_y)
  Parking/3(reversing) -> Reversing Coeff/1
  Parking Spot/1 -> Parking/3(parking_spot)
  Demux2/1 -> Parking/1(ev_x)
  Parking/4(turn) -> Turn Coeff/1
  Position/1 -> Demux2/1
  Parking/5(states) -> State/1
  Radians to Degrees/1 -> Parking/6(ev_yaw)
  Command/1 -> Parking/5(park_request), Compare To Constant/1

== system full_sim123deleteme/EV3/Position Control/State Integrators With Resets ==
  Position Set : Inport
  dx : Inport  Port=2
  dy : Inport  Port=3
  dtheta : Inport  Port=4
  Compare To Constant : simulink/Logic and Bit Operations/Compare To Constant  relop=>  const=0  OutDataTypeStr=boolean
  Constant1 : Constant  Value=[-0.39, 0.33, pi]
  Mux1 : Mux  Inputs=3
  Selector : Selector  InputPortWidth=4  IndexOptions=Index vector (dialog)  Indices=[2:4]  OutputSizes=1
  Selector1 : Selector  InputPortWidth=4  IndexOptions=Index vector (dialog)  Indices=1  OutputSizes=1
  Switch3 : Switch  Criteria=u2 ~= 0
  x1 : Integrator  ExternalReset=rising  InitialConditionSource=external  InitialCondition=initX
  Out2 : Outport
  wires:
  x1/1 -> Out2/1
  Mux1/1 -> x1/1
  Switch3/1 -> x1/3
  Constant1/1 -> Switch3/3
  Selector/1 -> Switch3/1
  dx/1 -> Mux1/1
  dtheta/1 -> Mux1/3
  dy/1 -> Mux1/2
  Selector1/1 -> Compare To Constant/1
  Compare To Constant/1 -> Switch3/2, x1/2
  Position Set/1 -> Selector/1, Selector1/1

== system full_sim123deleteme/EV3/Task Controls/Line Following PID ==
  RLI Error : Inport
  Derivative : Derivative
  Integrator : Integrator
  Kb : Gain  Gain=0
  Kd : Gain  Gain=0.005
  Ki : Gain  Gain=0
  Kp : Gain  Gain=0.1
  Saturation : Saturate  UpperLimit=15  LowerLimit=-15
  Sum : Sum  Inputs=+++
  Sum1 : Sum  Inputs=|++
  Sum2 : Sum  Inputs=-+|
  Steering : Outport
  wires:
  Sum/1 -> Sum2/1, Saturation/1
  Kd/1 -> Derivative/1
  Kp/1 -> Sum/1
  Integrator/1 -> Sum/2
  RLI Error/1 -> Kd/1, Ki/1, Kp/1
  Derivative/1 -> Sum/3
  Saturation/1 -> Sum2/2, Steering/1
  Ki/1 -> Sum1/1
  Sum1/1 -> Integrator/1
  Kb/1 -> Sum1/2
  Sum2/1 -> Kb/1

== system full_sim123deleteme/EV3/Task Controls/Motors ==
  note: Left Motor
  note: Right Motor
  Right Motor % : Inport
  Left Motor % : Inport  Port=2
  DC Motor (w/ load) 1 : Subsystem
  DC Motor (w/ load) 2 : Subsystem
  Gain : Gain  Gain=0.1
  Gain1 : Gain  Gain=0.1
  Right ω : Outport
  Left ω : Outport  Port=2
  wires:
  Gain1/1 -> DC Motor (w/ load) 2/1(va)  "var"
  DC Motor (w/ load) 2/1(ω) -> Right ω/1  "ωr"
  Gain/1 -> DC Motor (w/ load) 1/1(va)  "val"
  DC Motor (w/ load) 1/1(ω) -> Left ω/1  "ωl"
  Left Motor %/1 -> Gain/1
  Right Motor %/1 -> Gain1/1

== system full_sim123deleteme/EV3/Task Controls/Platoon PID ==
  Distance Error : Inport
  Derivative : Derivative
  Integrator : Integrator
  Kd : Gain  Gain=0
  Ki : Gain  Gain=0.02
  Kp : Gain  Gain=7
  Sum : Sum  Inputs=+++
  Platoon Speed : Outport
  wires:
  Sum/1 -> Platoon Speed/1
  Kd/1 -> Derivative/1
  Kp/1 -> Sum/1
  Ki/1 -> Integrator/1
  Integrator/1 -> Sum/2
  Distance Error/1 -> Kd/1, Ki/1, Kp/1
  Derivative/1 -> Sum/3

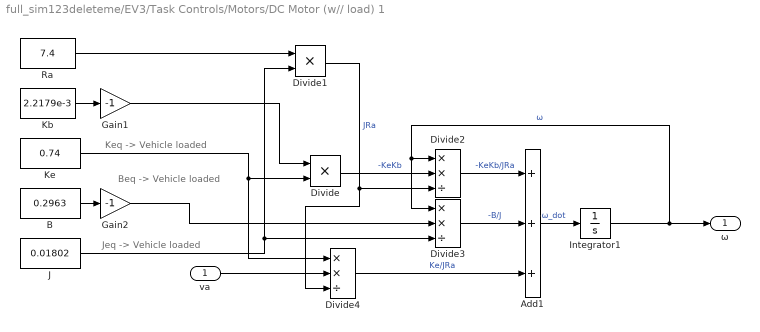
== system full_sim123deleteme/EV3/Task Controls/Motors/DC Motor (w// load) 1 ==
  note: Keq -> Vehicle loaded
  note: Jeq -> Vehicle loaded
  note: Beq -> Vehicle loaded
  va : Inport
  Add1 : Sum  Inputs=+++
  B : Constant  Value=0.2963
  Divide : Product  Inputs=**
  Divide1 : Product  Inputs=**
  Divide2 : Product  Inputs=**/
  Divide3 : Product  Inputs=**/
  Divide4 : Product  Inputs=**/
  Gain1 : Gain  Gain=-1
  Gain2 : Gain  Gain=-1
  Integrator1 : Integrator
  J : Constant  Value=0.01802
  Kb : Constant  Value=2.2179e-3
  Ke : Constant  Value=0.74
  Ra : Constant  Value=7.4
  ω : Outport
  wires:
  Divide2/1 -> Add1/1  "-KeKb/JRa"
  Divide3/1 -> Add1/2  "-B/J"
  Ra/1 -> Divide1/1
  Kb/1 -> Gain1/1
  Ke/1 -> Divide4/1, Divide/2
  J/1 -> Divide1/2, Divide3/3
  B/1 -> Gain2/1
  Gain2/1 -> Divide3/2
  Add1/1 -> Integrator1/1  "ω_dot"
  va/1 -> Divide4/2
  Gain1/1 -> Divide/1
  Divide/1 -> Divide2/2  "-KeKb"
  Divide1/1 -> Divide2/3, Divide4/3  "JRa"
  Divide4/1 -> Add1/3  "Ke/JRa"
  Integrator1/1 -> Divide3/1, Divide2/1, ω/1  "ω"

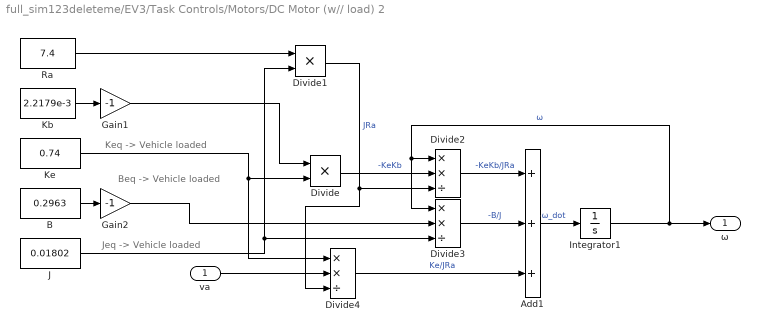
== system full_sim123deleteme/EV3/Task Controls/Motors/DC Motor (w// load) 2 ==
  note: Keq -> Vehicle loaded
  note: Jeq -> Vehicle loaded
  note: Beq -> Vehicle loaded
  va : Inport
  Add1 : Sum  Inputs=+++
  B : Constant  Value=0.2963
  Divide : Product  Inputs=**
  Divide1 : Product  Inputs=**
  Divide2 : Product  Inputs=**/
  Divide3 : Product  Inputs=**/
  Divide4 : Product  Inputs=**/
  Gain1 : Gain  Gain=-1
  Gain2 : Gain  Gain=-1
  Integrator1 : Integrator
  J : Constant  Value=0.01802
  Kb : Constant  Value=2.2179e-3
  Ke : Constant  Value=0.74
  Ra : Constant  Value=7.4
  ω : Outport
  wires:
  Divide2/1 -> Add1/1  "-KeKb/JRa"
  Divide3/1 -> Add1/2  "-B/J"
  Ra/1 -> Divide1/1
  Kb/1 -> Gain1/1
  Ke/1 -> Divide4/1, Divide/2
  J/1 -> Divide1/2, Divide3/3
  B/1 -> Gain2/1
  Gain2/1 -> Divide3/2
  Add1/1 -> Integrator1/1  "ω_dot"
  va/1 -> Divide4/2
  Gain1/1 -> Divide/1
  Divide/1 -> Divide2/2  "-KeKb"
  Divide1/1 -> Divide2/3, Divide4/3  "JRa"
  Divide4/1 -> Add1/3  "Ke/JRa"
  Integrator1/1 -> Divide3/1, Divide2/1, ω/1  "ω"

== matlab function full_sim123deleteme/Optitrack Simulation/MATLAB Function ==
  data: ev1pos input; packet output size=272; ev2pos input
function packet = fcn(ev1pos, ev2pos)
evs = {ev1pos,ev2pos};

packet = zeros(272,1,'uint8');

packet(1:2) = typecast(int16(7), 'uint8'); % packet type 
packet(17:20) = typecast(int32(length(evs)), 'uint8'); % num rigid bodies

for i = 1:length(evs)
    ptr = 21 + ((i-1)*120);
    pos = evs{i};
    q = eul2quat([pos(3),0,0]);
    % x, y, z, qx, qy, qz, qw
    packet(ptr+4:ptr+31) = typecast(single([pos(1) 0 pos(2) q(2) q(4) q(3) q(1)]), 'uint8');
end

== matlab function full_sim123deleteme/Unit Conversion/MATLAB Function1 ==
  data: u input; y output
function y = fcn(u)
% Converts from infinite degrees to +/-180 degrees yaw
    new_angle = mod(u, 360);
    if new_angle > 180.0
        new_angle = new_angle - 360.0;
    end
    y = new_angle;
end

== matlab function full_sim123deleteme/EV3/Localization and UI Control/Drive Selector/MATLAB Function ==
  data: deg_in input; deg_out output
function deg_out = remainder(deg_in)

deg_out = mod(deg_in+180,360)-180;

== matlab function full_sim123deleteme/EV3/Localization and UI Control/Drive Selector/MATLAB Function1 ==
  data: parking_spot_num input; act_deg output; states input; position input
function act_deg = atan_me(parking_spot_num, states, position)

if parking_spot_num ==1 && states == 10
    degg = atan2(1.8-position(2), 0-position(1)); 
    
elseif parking_spot_num ==2 && states ==10
    degg = atan2(1.525 - position(2), 0-position(1));
    
elseif parking_spot_num ==3 && states == 10
    degg = atan2(1.1 - position(2), 0-position(1));
    
elseif parking_spot_num == 1 && states == 20
    %go to parking spot 1
    degg= atan2(1.6-position(2), -0.45-position(1)); 
%     degg = -168;
    
elseif parking_spot_num ==2 && states == 20
     %go to parking spot 2
    degg =atan2(1.2-position(2), -0.75-position(1)); 
%     degg = -165;
    
elseif parking_spot_num ==3 && states == 20 
    %go to parkin spot 3
    degg = atan2(0.80-position(2), -0.85-position(1)); 
%     degg = -150;
elseif parking_spot_num ~=0 && states == 30
    %complete parking and move angle to 180 degrees
    degg = pi; 
    
elseif parking_spot_num ~=0 && states == 40 
    %go to stop sign
    degg = atan2(0.525-position(2),0.0935-position(1)); 
    
elseif parking_spot_num ~=0 && states == 50
    degg = atan2(0.33 - position(2), -0.3 - position(1));
    %degg = -90; 
    
else
    degg = 0;
end 
act_deg = rad2deg(degg);
%act_deg = degg;

== matlab function full_sim123deleteme/EV3/Localization and UI Control/Head Turning/MATLAB Function ==
  data: headTarget input; angle output; position input
function angle = headAngle(headTarget, position)

diff = headTarget - position(1:2);
angle = -double(rad2deg(atan2(diff(2),diff(1))-position(3)));
angle = mod(angle+180, 360) - 180;

== matlab function full_sim123deleteme/EV3/Localization and UI Control/Localization/MATLAB Function ==
  data: dx output; dist input; angle input; dy output
function [dx,dy] = arc_approximation(dist,angle)
    if angle == 0
        dx = dist;
        dy = 0;
    else
        dx = sin(angle) * dist / angle;
        dy = (1-cos(angle)) * dist / angle;
    end

== matlab function full_sim123deleteme/EV3/Localization and UI Control/Localization/MATLAB Function1 ==
  data: x input; x output; y input; r input; y output
function [x,y] = rotate2d(x,y,r)
    rot = [cos(r) -sin(r); sin(r) cos(r)] * [x;y];
    x = rot(1);
    y = rot(2);

== matlab function full_sim123deleteme/EV3/Localization and UI Control/MATLAB Function ==
  data: right output; speed input; left output; steering input
function [right, left]= toMotorSpeeds(speed, steering)

left = speed - steering;
right = speed + steering;

m = max(left,right);
if m > 100
    left = left - m + 100;
    right = right - m + 100;
end

== matlab function full_sim123deleteme/EV3/Localization and UI Control/Optitrack Receive//Filter/MATLAB Function ==
  data: data input; new input; arr input; valid output boolean; arr output
function [valid, arr]= filter(data,new,arr)

valid = false;
if new
    arr = circshift(arr,1);
    arr(1) = data(3);
    d = diff(arr);
    d = d - 2*pi*round(d/(2*pi));
    valid = all(abs(d) < deg2rad(5), 'all');
end

== stateflow chart full_sim123deleteme/EV3/Localization and UI Control/Stateflow/Parking ==
  settings: executeAtInitialization=1
  state Leader_Goto_Intersection
    entry:
    linetracking =1;
    platooning =0;
    reversing = 0;
    turn = 0;
    stop =0;
    states = 10000;
  state Follower_Goto_Intersection
    entry:
    linetracking = 0;
    platooning =1;
    reversing = 0;
    turn =0;
    stop =0;
    states = 01000;
  state Enter_ParkingArea
    %Turn car 90 degrees
    entry:
    linetracking = 0;
    platooning =0;
    reversing = 0;
    turn = -1;
    stop =0;
    states = 00010;
  state Find_ParkingSpot
    entry:
    linetracking = 0;
    platooning  =0;
    reversing = 0;
    turn =2;
    stop = 0;
    states = 00020;
    %turn = 2 means find park (step 2 in turning)
    %Use the center of the target values to solve for the desired yaw that we want
    % Parking Spot 1 : x_cent = -0.45 ; y_cent =  1.6
    %Parking Spot 2: x_cent = -0.75; y_cent = 1.2
    %Parking Spot 3: x_cent = -0.85; y_cent = 0.80
  state Parking
    entry:
    linetracking = 0;
    platooning = 0;
    reversing = 0;
    turn=3;
    stop = 0;
    states = 00030;
    %turn =3 means 180 degrees
    %parking means to slow down the motor speed,
    %and to use ultrasonic sensor to detect for wall to stop
    %If ultrasonic sensor reaches a range of values-->parked
  state Parked
    entry:
    linetracking = 0;
    platooning = 0;
    reversing = 0;
    turn=0;
    stop = 1;
    states = 00001;
    %stop the car
  state Manual_Control
    entry:
    manual_control = 1;
    states = 100000;
    exit:
    manual_control = 0;
  state Reverse_Out_Spot
    entry:
    linetracking = 0;
    platooning = 0;
    reversing = 1;
    turn = 0;
    stop = 0;
    states = 00100;
    %once we find coordinate spot b we can
    %get rid of line tracking
  state Goto_Stop_Sign
    entry:
    linetracking = 0;
    platooning =0;
    reversing = 0;
    turn = 4;
    stop = 0;
    states = 00040;
    %turn = 4 means parking sign angle
  state Turn_Car_toInter
    %turn car -90 degrees
    entry:
    linetracking = 0;
    platooning =0;
    reversing = 0;
    turn = 5;
    stop = 0;
    states = 00050;
  state Finished
    entry:
    linetracking = 1;
    platooning =0;
    reversing = 0;
    turn =0;
    stop = 0;
    states = 10000;
    %can continue to linetrack the path.
  Manual_Control -> Leader_Goto_Intersection : [park_request ~= 4]
  Finished -> Leader_Goto_Intersection [order 1]
  (default) -> Leader_Goto_Intersection
  Leader_Goto_Intersection -> Follower_Goto_Intersection [order 1] : [park_request ==2]
  Leader_Goto_Intersection -> Manual_Control [order 3] : [park_request == 4]
  Follower_Goto_Intersection -> Manual_Control [order 3] : [park_request == 4]
  Follower_Goto_Intersection -> Leader_Goto_Intersection [order 1] : [park_request ==1]
  Leader_Goto_Intersection -> Enter_ParkingArea [order 2] : [park_request == 3 && ev_x <= 0.2 && ev_x >= -0.2...
      |  && ev_y <=3 && ev_y >= 2 ]
  Follower_Goto_Intersection -> Enter_ParkingArea [order 2] : [park_request == 3 && ev_x <= 0.2 && ev_x >= -0.2...
      |  && ev_y <=3 && ev_y >= 2 ]
  Enter_ParkingArea -> Manual_Control [order 2] : [park_request == 4]
  Enter_ParkingArea -> Find_ParkingSpot [order 1] : [(ev_yaw <=-85 && ev_yaw>= -95)&&...
      | ((parking_spot ==1 && ev_x <=0.30 && ev_x >=-0.30 && ev_y<=1.9 && ev_y >= 1.7) ||...
      |  (parking_spot == 2 && ev_x <= 0.30 && ev_x>= -0.30 && ev_y<=1.6 && ev_y >= 1.45) ||...
      |  (parking_spot ==3 && ev_x <=0.30&& ev_x >= -0.30 && ev_y <=1.2 && ev_y >= 1))]
  Find_ParkingSpot -> Manual_Control [order 2] : [park_request == 4]
  Find_ParkingSpot -> Parking [order 1] : [(parking_spot ==1 && ev_x <= -0.40 && ev_x >= -0.50 && ev_y<=1.7...
      |  && ev_y >= 1.5) || (parking_spot == 2 && ev_x<=-0.70 && ev_x>=-0.80....
      |  && ev_y<=1.3 && ev_y >= 1.1) || (parking_spot ==3 ...
      | && ev_x <=-0.80 && ev_x>= -0.90 && ev_y>=0.70 && ev_y <=0.90)]
  Parking -> Manual_Control [order 2] : [park_request == 4]
  Parking -> Parked [order 1] : [Ultrasonic <= 15]
  Parked -> Manual_Control [order 2] : [park_request == 4]
  Parked -> Reverse_Out_Spot [order 1] : [park_request == 1 || park_request ==2]
  Turn_Car_toInter -> Manual_Control [order 2] : [park_request == 4]
  Goto_Stop_Sign -> Manual_Control [order 2] : [park_request == 4]
  Finished -> Manual_Control [order 2] : [park_request == 4]
  Reverse_Out_Spot -> Manual_Control [order 2] : [park_request == 4]
  Reverse_Out_Spot -> Goto_Stop_Sign [order 1] : [(parking_spot ==1 && ev_x <=0.30 && ev_x >=-0.30 ...
      | && ev_y<=1.9 && ev_y >= 1.4) || (parking_spot == 2 ...
      |   && ev_x <= 0.30 && ev_x>= -0.30 && ev_y<=1.3 ...
      | && ev_y >= 1) || (parking_spot ==3 && ev_x <=0.30...
      | && ev_x >= -0.30 && ev_y <=1 && ev_y >= 0.65)]
  Goto_Stop_Sign -> Turn_Car_toInter [order 1] : [ev_x <= 0.17 && ev_x >= 0.017...
      |  && ev_y >= 0.45 && ev_y <= 0.6]
  Turn_Car_toInter -> Finished [order 1] : [ev_x>=-0.5 && ev_x <= -0.10 && ev_y<=0.36 && ev_y >= 0.3 ]
  data: ev_x input; ev_y input; parking_spot input; Ultrasonic input; linetracking output double; stop output double; reversing output double; turn output double; states output double; park_request input; ev_yaw input; platooning output double; manual_control output double
